simulink model "two_fsk_2"  (R2021a)
settings: Solver=VariableStepAuto  StartTime=0.0  StopTime=10.0  RelTol=1e-3
settings Model: Creator=27734  LastModifiedBy=27734

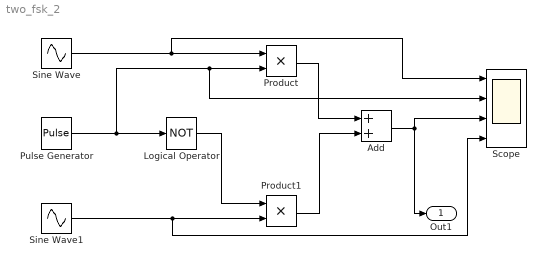
== system two_fsk_2 ==
  Add : Sum
  Logical Operator : Logic  Operator=NOT  AllPortsSameDT=off  OutDataTypeStr=boolean
  Product : Product
  Product1 : Product
  Pulse Generator : DiscretePulseGenerator  PulseType=Time based  Period=3  PulseWidth=33
  Scope : Scope  NumInputPorts=4
  Sine Wave : Sin  Frequency=20*pi  SampleTime=0.002
  Sine Wave1 : Sin  Frequency=120*pi  SampleTime=0.002
  Out1 : Outport
  wires:
  Logical Operator/1 -> Product1/1
  Add/1 -> Out1/1, Scope/3
  Product/1 -> Add/1
  Product1/1 -> Add/2
  Sine Wave1/1 -> Scope/4, Product1/2
  Sine Wave/1 -> Scope/1, Product/1
  Pulse Generator/1 -> Scope/2, Product/2, Logical Operator/1
